simulink model "Pacejka_Tyre_Model_2023b"  (R2023b)
settings: Solver=FixedStepAuto  StartTime=0.0  StopTime=1  FixedStep=0.005  MinStep=1e-1  RelTol=1e-3
PreLoadFcn:
  | % Adding to path the location of .slx file:
  | addpath(fileparts(get_param(bdroot,'FileName')));
  | 
  | % init values:
  | pacajeka_init;
values from neighbouring files (symbols this model uses):
  a0 = 1.6    [pacajeka_init.m]    (also in pacajeka_model_param.mat)
  a1 = -34    [pacajeka_init.m]    (also in pacajeka_model_param.mat)
  a2 = 1250    [pacajeka_init.m]    (also in pacajeka_model_param.mat)
  a3 = 2320    [pacajeka_init.m]    (also in pacajeka_model_param.mat)
  a4 = 12.8    [pacajeka_init.m]    (also in pacajeka_model_param.mat)
  a5 = 0    [pacajeka_init.m]    (also in pacajeka_model_param.mat)
  a6 = -0.0053    [pacajeka_init.m]    (also in pacajeka_model_param.mat)
  a7 = 0.1925    [pacajeka_init.m]    (also in pacajeka_model_param.mat)
  a8 = 0    [pacajeka_init.m]    (also in pacajeka_model_param.mat)
  b0 = 1.55    [pacajeka_init.m]    (also in pacajeka_model_param.mat)
  b1 = 0    [pacajeka_init.m]    (also in pacajeka_model_param.mat)
  b2 = 1000    [pacajeka_init.m]    (also in pacajeka_model_param.mat)
  b3 = 60    [pacajeka_init.m]    (also in pacajeka_model_param.mat)
  b4 = 300    [pacajeka_init.m]    (also in pacajeka_model_param.mat)
  b5 = 0.17    [pacajeka_init.m]    (also in pacajeka_model_param.mat)
  b6 = 0    [pacajeka_init.m]    (also in pacajeka_model_param.mat)
  b7 = 0    [pacajeka_init.m]    (also in pacajeka_model_param.mat)
  b8 = 0.2    [pacajeka_init.m]    (also in pacajeka_model_param.mat)
CloseFcn:
  | % clearing the path
  | rmpath(fileparts(get_param(bdroot,'FileName')));
settings Model: Creator=Milosh Yokich  LastModifiedBy=Milosh Yokich
settings DataIOCC: ExternalInput=ds  LoadExternalInput=on

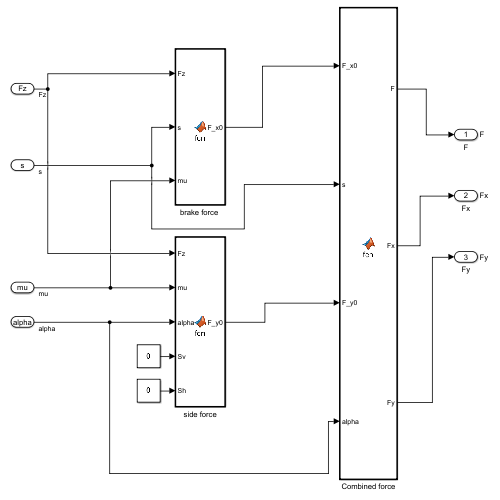
[thumbnail: Simulink's stored preview of the top-level diagram]
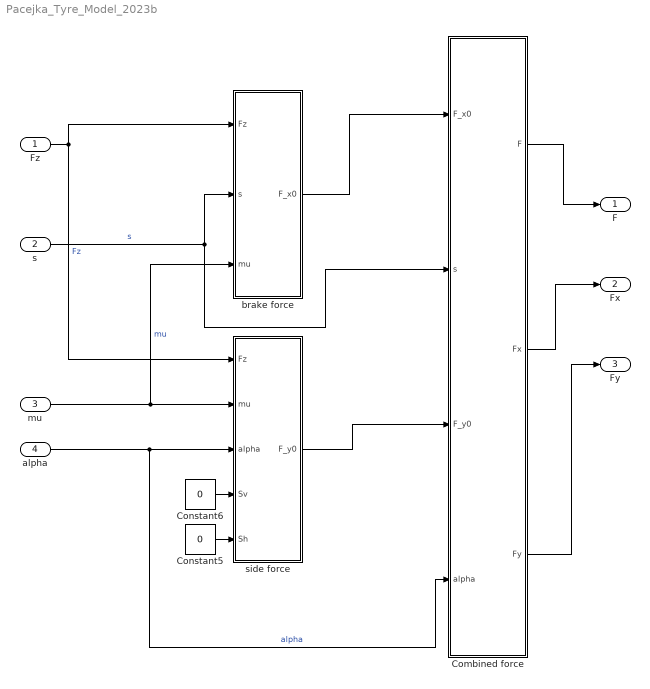
== system Pacejka_Tyre_Model_2023b ==
  Fz : Inport
  s : Inport  Port=2
  mu : Inport  Port=3
  alpha : Inport  Port=4
  Combined force : MATLAB Function  TreatAsAtomicUnit=on
  Constant5 : Constant  Value=0
  Constant6 : Constant  Value=0
  "brake force " : MATLAB Function  TreatAsAtomicUnit=on
  side force : MATLAB Function  TreatAsAtomicUnit=on
  F : Outport  SignalName=F
  Fx : Outport  Port=2  SignalName=Fx
  Fy : Outport  Port=3  SignalName=Fy
  wires:
  Fz/1 -> "brake force "/1(Fz), side force/1(Fz)  "Fz"
  Constant6/1 -> side force/4(Sv)
  Constant5/1 -> side force/5(Sh)
  "brake force "/1(F_x0) -> Combined force/1(F_x0)
  side force/1(F_y0) -> Combined force/3(F_y0)
  s/1 -> Combined force/2(s), "brake force "/2(s)  "s"
  mu/1 -> "brake force "/3(mu), side force/2(mu)  "mu"
  alpha/1 -> Combined force/4(alpha), side force/3(alpha)  "alpha"
  Combined force/1(F) -> F/1
  Combined force/2(Fx) -> Fx/1
  Combined force/3(Fy) -> Fy/1

== matlab function Pacejka_Tyre_Model_2023b/side force ==
  data: Fz input; mu input; alpha input; Sv input; Sh input; F_y0 output; a0 parameter; a1 parameter; a2 parameter; a3 parameter; a4 parameter; a6 parameter; a7 parameter; a5 parameter; a8 parameter
function F_y0 = fcn(Fz, mu, alpha, Sv, Sh, a0, a1, a2, a3, a4, a6, ...
    a7, a5, a8)
persistent C D B E

% init persistent variables: 
if isempty(C)
    C = a0;
    D = mu*(a1*Fz^2 + a2*Fz);
    B = (a3*sin(2*atan(Fz/a4)))/C/D;
    E = a6*Fz +a7;

end
X = alpha + Sh;
F_y0 = -(D*sin(C*atan(B*((1-E)*X + E/B*atan(B*X)))) + Sv);

== matlab function Pacejka_Tyre_Model_2023b/brake force  ==
  data: Fz input; s input; mu input; F_x0 output; b0 parameter; b1 parameter; b2 parameter; b3 parameter; b4 parameter; b6 parameter; b7 parameter; b5 parameter; b8 parameter
function F_x0 = fcn(Fz, s, mu, b0, b1, b2, b3, b4, b6, b7, b5, b8)
persistent C D B E

% init persistent variables: 
if isempty(C)
    C = b0;
    D = mu*(b1*Fz^2 + b2*Fz);
    B = (b3*Fz^2 + b4*Fz)/(C*D*exp(b5*Fz));
    E = b6*Fz^2 + b7*Fz + b8;

end
X = s;
F_x0 = (D*sin(C*atan(B*((1-E)*X + E/B*atan(B*X)))));

== matlab function Pacejka_Tyre_Model_2023b/Combined force ==
  data: F_x0 input; F output; s input; F_y0 input; alpha input; Fx output; Fy output
 function [F, Fx, Fy] = fcn(F_x0, s, F_y0, alpha)


% normalization of s
s = s/100;
alpha_rad = alpha/180*pi;

beta = atan2(sin(alpha_rad), s);

Fx = F_x0*abs(cos(beta));

Fy = F_y0*abs(sin(beta));

F =  F_x0*cos(beta)^2 + F_y0*sin(beta)^2;
